simulink model "fig2_17"  (Simulink 8.1)
settings: Solver=ode45  StartTime=0.0  StopTime=10.0  MaxStep=.05  MinStep=.01  RelTol=1e-3
settings Model: Creator=Office Depot  LastModifiedBy=David Powell
settings SolverCC: InitialStep=.01
settings OptimizationCC: InitFltsAndDblsToZero=on
settings DebuggingCC: StrictBusMsg=Warning

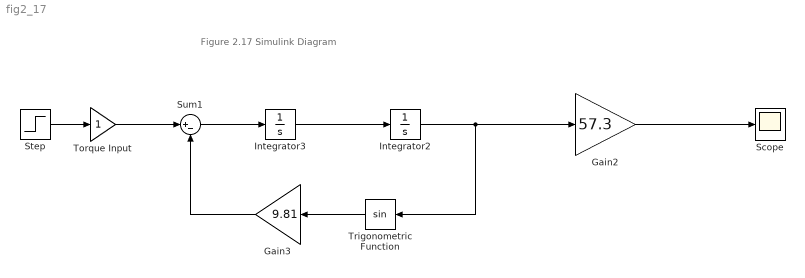
== system fig2_17 ==
  note: Figure 2.17 Simulink Diagram
  Gain2 : Gain  Gain=57.3
  Gain3 : Gain  Gain=9.81
  Integrator2 : Integrator
  Integrator3 : Integrator
  Scope : Scope
  Step : Step  SampleTime=0
  Sum1 : Sum  Inputs=|+-
  Torque Input : Gain
  Trigonometric Function : Trigonometry
  wires:
  Step/1 -> Torque Input/1
  Torque Input/1 -> Sum1/1
  Integrator2/1 -> Trigonometric Function/1, Gain2/1
  Integrator3/1 -> Integrator2/1
  Sum1/1 -> Integrator3/1
  Gain2/1 -> Scope/1
  Trigonometric Function/1 -> Gain3/1
  Gain3/1 -> Sum1/2
